simulink model "Park_Test"  (R2022a)
settings: Solver=VariableStepAuto  StartTime=0.0  StopTime=10.0  RelTol=1e-3
libraries: MyPMSMLibrary x1
settings Model: Creator=jff_1  LastModifiedBy=jff_1

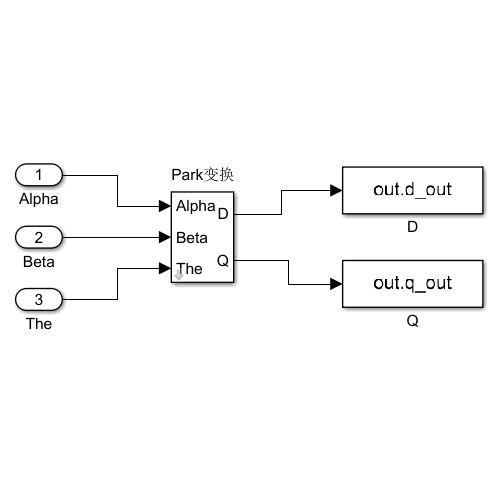
[thumbnail: Simulink's stored preview of the top-level diagram]
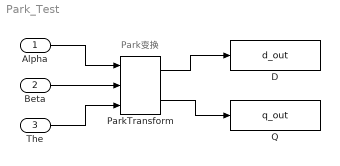
== system Park_Test ==
  note: Park变换
  Alpha : Inport
  Beta : Inport  Port=2
  The : Inport  Port=3
  D : ToWorkspace  VariableName=d_out  SampleTime=-1
  ParkTransform : MyPMSMLibrary/Transforms/ParkTransform
  Q : ToWorkspace  VariableName=q_out  SampleTime=-1
  wires:
  Alpha/1 -> ParkTransform/1
  Beta/1 -> ParkTransform/2
  The/1 -> ParkTransform/3
  ParkTransform/1 -> D/1
  ParkTransform/2 -> Q/1
